simulink model "DCMtoAxisAngleSubsystem"  (R2024a)
settings: Solver=VariableStepAuto  StartTime=0.0  StopTime=10.0  RelTol=1e-3
settings Model: Creator=Spencer  LastModifiedBy=Spencer

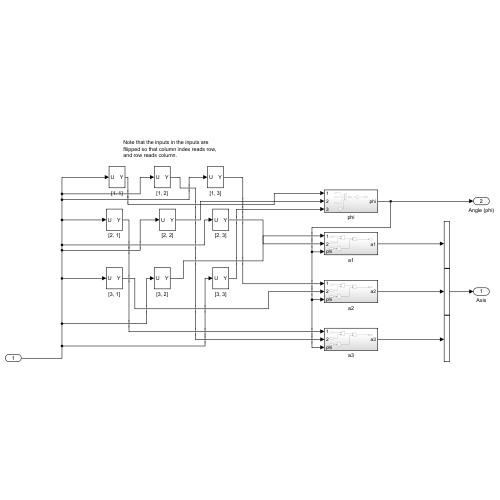
[thumbnail: Simulink's stored preview of the top-level diagram]
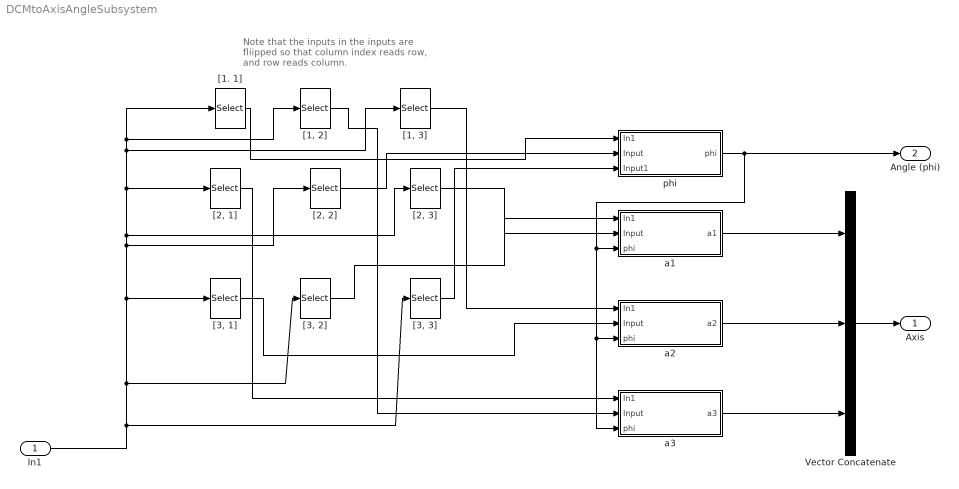
== system DCMtoAxisAngleSubsystem ==
  note: Note that the inputs in the inputs are fliipped so that column index reads row, and row reads column.
  In1 : Inport
  Vector Concatenate : Concatenate  NumInputs=3
  "[1, 2]" : Selector  NumberOfDimensions=2  InputPortWidth=3  IndexOptions=Index vector (dialog),Index vector (dialog)  Indices=2,1  OutputSizes=1,1
  "[1, 3]" : Selector  NumberOfDimensions=2  InputPortWidth=3  IndexOptions=Index vector (dialog),Index vector (dialog)  Indices=3,1  OutputSizes=1,1
  "[1. 1]" : Selector  NumberOfDimensions=2  InputPortWidth=3  IndexOptions=Index vector (dialog),Index vector (dialog)  Indices=1,1  OutputSizes=1,1
  "[2, 1]" : Selector  NumberOfDimensions=2  InputPortWidth=3  IndexOptions=Index vector (dialog),Index vector (dialog)  Indices=1,2  OutputSizes=1,1
  "[2, 2]" : Selector  NumberOfDimensions=2  InputPortWidth=3  IndexOptions=Index vector (dialog),Index vector (dialog)  Indices=2,2  OutputSizes=1,1
  "[2, 3]" : Selector  NumberOfDimensions=2  InputPortWidth=3  IndexOptions=Index vector (dialog),Index vector (dialog)  Indices=3,2  OutputSizes=1,1
  "[3, 1]" : Selector  NumberOfDimensions=2  InputPortWidth=3  IndexOptions=Index vector (dialog),Index vector (dialog)  Indices=1,3  OutputSizes=1,1
  "[3, 2]" : Selector  NumberOfDimensions=2  InputPortWidth=3  IndexOptions=Index vector (dialog),Index vector (dialog)  Indices=2,3  OutputSizes=1,1
  "[3, 3]" : Selector  NumberOfDimensions=2  InputPortWidth=3  IndexOptions=Index vector (dialog),Index vector (dialog)  Indices=3,3  OutputSizes=1,1
  a1 : Subsystem
  a2 : Subsystem
  a3 : Subsystem
  phi : Subsystem
  Axis : Outport
  Angle (phi) : Outport  Port=2
  wires:
  "[1. 1]"/1 -> phi/1(In1)
  a1/1(a1) -> Vector Concatenate/1
  "[3, 1]"/1 -> a2/2(Input)
  a2/1(a2) -> Vector Concatenate/2
  Vector Concatenate/1 -> Axis/1
  a3/1(a3) -> Vector Concatenate/3
  "[2, 1]"/1 -> a3/1(In1)
  In1/1 -> "[3, 2]"/1, "[3, 1]"/1, "[2, 1]"/1, "[1, 3]"/1, "[1, 2]"/1, "[1. 1]"/1, "[2, 3]"/1, "[2, 2]"/1, "[3, 3]"/1
  "[2, 3]"/1 -> a1/2(Input)
  "[1, 3]"/1 -> a2/1(In1)
  "[3, 3]"/1 -> phi/3(Input1)
  "[2, 2]"/1 -> phi/2(Input)
  phi/1(phi) -> a3/3(phi), a2/3(phi), a1/3(phi), Angle (phi)/1
  "[3, 2]"/1 -> a1/1(In1)
  "[1, 2]"/1 -> a3/2(Input)

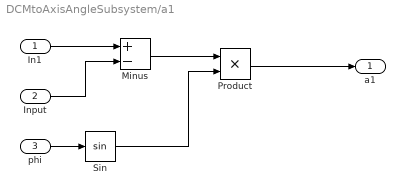
== system DCMtoAxisAngleSubsystem/a1 ==
  In1 : Inport
  Input : Inport  Port=2
  phi : Inport  Port=3
  Minus : Sum  Inputs=+-
  Product : Product
  Sin : Trigonometry
  a1 : Outport
  wires:
  In1/1 -> Minus/1
  Input/1 -> Minus/2
  phi/1 -> Sin/1
  Sin/1 -> Product/2
  Minus/1 -> Product/1
  Product/1 -> a1/1

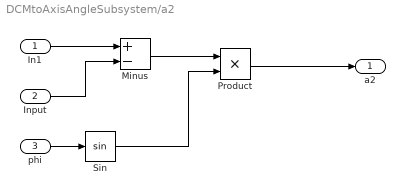
== system DCMtoAxisAngleSubsystem/a2 ==
  In1 : Inport
  Input : Inport  Port=2
  phi : Inport  Port=3
  Minus : Sum  Inputs=+-
  Product : Product
  Sin : Trigonometry
  a2 : Outport
  wires:
  In1/1 -> Minus/1
  Input/1 -> Minus/2
  phi/1 -> Sin/1
  Sin/1 -> Product/2
  Minus/1 -> Product/1
  Product/1 -> a2/1

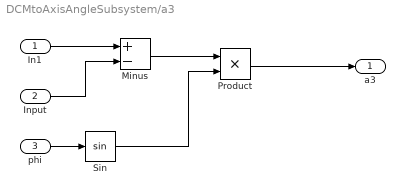
== system DCMtoAxisAngleSubsystem/a3 ==
  In1 : Inport
  Input : Inport  Port=2
  phi : Inport  Port=3
  Minus : Sum  Inputs=+-
  Product : Product
  Sin : Trigonometry
  a3 : Outport
  wires:
  In1/1 -> Minus/1
  Input/1 -> Minus/2
  phi/1 -> Sin/1
  Sin/1 -> Product/2
  Minus/1 -> Product/1
  Product/1 -> a3/1

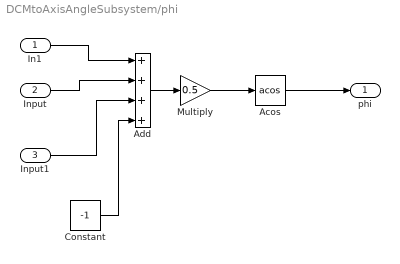
== system DCMtoAxisAngleSubsystem/phi ==
  In1 : Inport
  Input : Inport  Port=2
  Input1 : Inport  Port=3
  Acos : Trigonometry  Operator=acos
  Add : Sum  Inputs=++++
  Constant : Constant  Value=-1
  Multiply : Gain  Gain=0.5
  phi : Outport
  wires:
  Input1/1 -> Add/3
  Input/1 -> Add/2
  In1/1 -> Add/1
  Constant/1 -> Add/4
  Add/1 -> Multiply/1
  Multiply/1 -> Acos/1
  Acos/1 -> phi/1
